simulink model "PLANTA_CODESYS"  (R2024b)
settings: Solver=FixedStepAuto  StartTime=0.0  StopTime=inf  FixedStep=0.001  MaxStep=0.0005  RelTol=1e-4
undefined symbols (not defined in the file): A_hm, A_tm, at_breakpoints, b_ha, B_hm, b_ta, B_tm, bcx, bcy, bhd, bhEb, bhm, bt, btd, btm, btw, bwu, C_hm, C_tm, D_hm, D_tm, DiscIntNeverNeededParam, dl_h_ini, dx_l_ini, dx_t_ini, dx_td_ini, dxt_max, dy_l_ini, g, Hc, ih, it, J_eqt, Jhd_hEb, Jhm_hb, Jtd, Jtm_tb, K_hsa, K_hsia, K_tsa, K_tsia, Kcy, Kd_table, ke_int, Ke_tita, ke_tita, ke_w, Ke_w, kp_pos, Kp_table, kp_w, kpos, Ktw, kwu, l_breakpoints, l_h_ini, Lh0, ml_breakpoints, Ms, Mt ... (+16)
libraries: simulink x11, spsEdgeDetectorLib x5, simulink_extras x2, opcualib x2, dspsigops x2, dspstat3 x1, vrlib x1, sldrtlib x1
(part 1 of 2)
settings Model: Creator=ribei  LastModifiedBy=ribei
settings SolverCC: AllowMultiTaskInputOutput=on  ZeroCrossAlgorithm=Adaptive  AutoInsertRateTranBlk=on
settings DebuggingCC: IgnoredZcDiagnostic=none  UnderSpecifiedDimensionMsg=warning

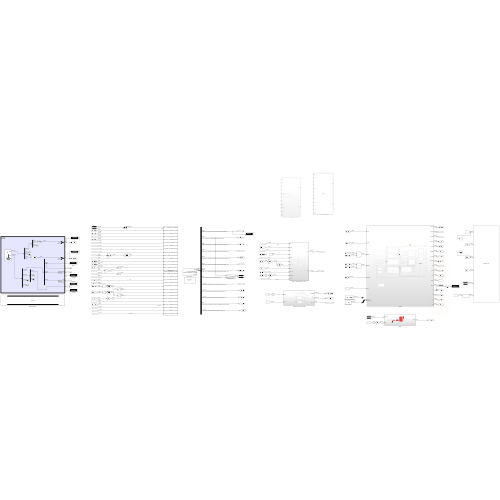
[thumbnail: Simulink's stored preview of the top-level diagram]
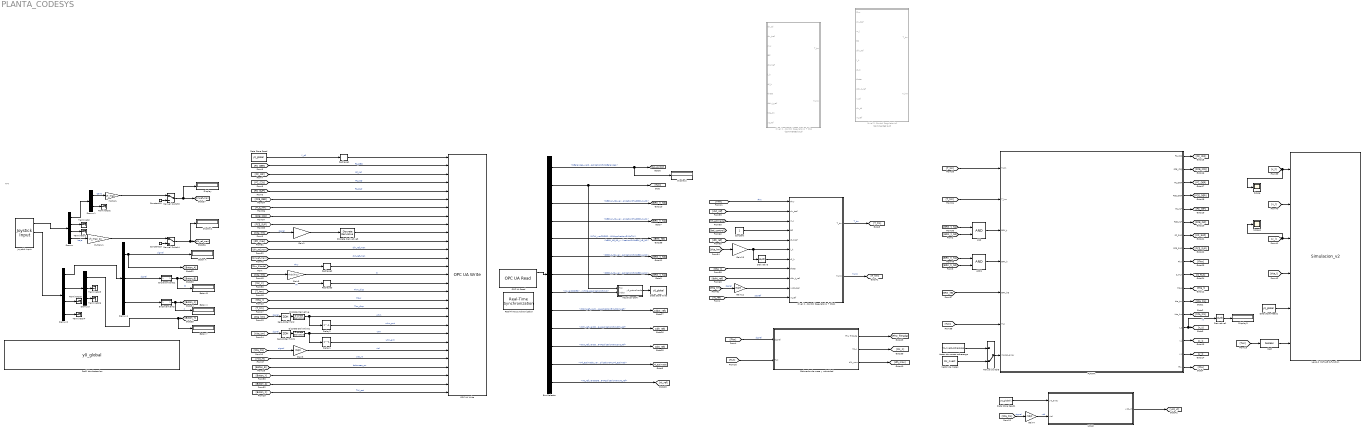
== system PLANTA_CODESYS ==
  note: HMI
  AND : Logic  IconShape=distinctive  AllPortsSameDT=off  OutDataTypeStr=boolean
  AND1 : Logic  IconShape=distinctive  AllPortsSameDT=off  OutDataTypeStr=boolean
  Actualizar perfil : Subsystem
  Boton A : Display
  Boton B : Display
  Boton X : Display
  Boton Y : Display
  Bus Selector : BusSelector  OutputSignals=bBalanceo_varCODESYSControlWinV3X64ApplicationGVLbBalanceo,bTLK_varCODESYSControlWinV3X64ApplicationGVLbTLK,bBRK_h_N0_varCODESYSControlWinV3X64ApplicationGVLbBRK_h_N0,bBRK_h_N1_varCODESYSControlWinV3X64ApplicationGVLbBRK_h_N1,bBRK_hE_N0_varCODESYSControlWinV3X64ApplicationGVLbBRK_hE_N0,bBRK_t_N0_varCODESYSControlWinV3X64ApplicationGVLbBRK_t_N0,bBRK_t_N1_varCODESYSControlWinV3X64ApplicationGVLbBRK_t_N1,iC_varCODESYSControlWinV3X64ApplicationGVLiC,rDdxt_ref_varCODESYSControlWinV3X64ApplicationGVLrDdxt_ref,rDlh_ref_varCODESYSControlWinV3X64ApplicationGVLrDlh_ref,rDxt_ref_varCODESYSControlWinV3X64ApplicationGVLrDxt_ref,rMl_estimada_varCODESYSControlWinV3X64ApplicationGVLrMl_estimad,rXt_ref_varCODESYSControlWinV3X64ApplicationGVLrXt_ref
  Cast : DataTypeConversion  OutDataTypeStr=boolean  SaturateOnIntegerOverflow=off  RndMeth=Floor
  Constant : Constant
  Constant18 : Constant  Value=0  SampleTime=T_s1
  Constant19 : Constant  Value=0  SampleTime=T_s1
  Data Store Read : DataStoreRead  DataStoreName=y0_global  IndexOptions=Index vector (dialog)  Indices=1  OutputSizes=1
  Data Store Read1 : DataStoreRead  DataStoreName=y0_global  DataStoreElements=y0_global(:)  IndexOptions=Index vector (dialog)  Indices=1  OutputSizes=1
  Data Store Read2 : DataStoreRead  DataStoreName=y0_global  IndexOptions=Index vector (dialog)  Indices=1  OutputSizes=1
  Data Store Write : DataStoreWrite  DataStoreName=y0_global  IndexOptions=Index vector (dialog)  Indices=1  OutputSizes=1
  Delay1 : Delay  DelayLength=1  InputProcessing=Columns as channels (frame based)  SampleTime=T_s1
  Delay2 : Delay  DelayLength=1  InputProcessing=Columns as channels (frame based)  SampleTime=T_s1
  Demux : Demux
  Demux1 : Demux  Outputs=2
  Demux2 : Demux
  Demux3 : Demux  Outputs=3
  Demux4 : Demux  Outputs=3
  Derivative : Derivative
  Derivative1 : Derivative
  Discrete Derivative : simulink/Discrete/Discrete Derivative  gainval=1.0  ICPrevScaledInput=0.0  OutMin=[]  OutMax=[]  OutDataType=fixdt(1, 16)  OutScaling=2^-10  DoSatur=off
  Discrete Derivative1 : simulink/Discrete/Discrete Derivative  gainval=1.0  ICPrevScaledInput=0.0  OutMin=[]  OutMax=[]  OutDataType=fixdt(1, 16)  OutScaling=2^-10  DoSatur=off
  Discrete Derivative3 : simulink/Discrete/Discrete Derivative  gainval=1.0  ICPrevScaledInput=0.0  OutMin=[]  OutMax=[]  OutDataType=fixdt(1, 16)  OutScaling=2^-10  DoSatur=off
  Display{,1..3} (4 alike) : Display
  Enclavamiento : Stateflow chart  TreatAsAtomicUnit=on
  Enclavamiento1 : Stateflow chart  TreatAsAtomicUnit=on
  Estimador de masa y velocidad : Subsystem
  Gain1 : Gain  Gain=-rhd/(ih*2)
  Gain12 : Gain  Gain=rtd/it
  Gain13 : Gain  Gain=-rhd/(ih*2)
  Gain3 : Gain  Gain=rtd/it
  Gain4 : Gain  Gain=rtd/it
  Gain5 : Gain  Gain=-rhd/(ih*2)
  Joystick Input : vrlib/Joystick Input  joyid=1  adjustports=on  forcefeed=off
  LIDAR : Subsystem
  Level-2 MATLAB S-Function : M-S-Function  FunctionName=Simulacion_v2  Parameters=2.438, 2.591, 1.500, 0.850, 0.750, 7.500, 2.100, 2.500, 'black', 'black', '#E99000', 5.000
  Manual Switch3 : ManualSwitch
  Manual Switch4 : ManualSwitch
  Manual Switch5 : ManualSwitch  CurrentSetting=0
  Multiply : Gain  Gain=vt_max
  Multiply1 : Gain  Gain=vh_max_sc
  Nivel 2 - Control Regulatorio + Obs : Subsystem  Commented=on
  Nivel 2 - Control Regulatorio + Obs1 : Subsystem
  Nivel 2: Control Regulatorio1 : MATLAB Function  Commented=on  TreatAsAtomicUnit=on  SystemSampleTime=T_s2
  OPC UA Read : opcualib/OPC UA Read  SelectedServer=OPCUAServer@DESKTOP-L47GKVF  ServerList=OPCUAServer@DESKTOP-L47GKVF  NodeList={ '1', 'bBalanceo', '4', '|var|CODESYS Control Win V3 x64.Application.GVL.bBalanceo', '0'; '2', 'bBRK_h_N0', '4', '|var|CODESYS Control Win V3 x64.Application.GVL.bBRK_h_N0', '0'; '3', 'bBRK_h_N1', '4', '|var|CODESYS Control Win V3 x64.Application.GVL.bBRK_h_N1', '0'; '4', 'bBRK_hE_N0', '4', '|var|CODESYS Control Win V3 x64.Application.GVL.bBRK_hE_N0', '0'; '5', 'bBRK_t_N0', '4', '|var|CODESYS Control Win V3 x64.Application.GVL.bBRK_t_N0', '0'; '6', 'bBRK_t_N1', '4', '|var|CODESYS Control Win V3 x64.Application.GVL.bBRK_t_N1', '0'; '7', 'bTLK', '4', '|var|CODESYS Control Win V3 x64.Application.GVL.bTLK', '0'; '8', 'iC', '4', '|var|CODESYS Control Win V3 x64.Application.GVL.iC', '0'; '9', 'rDdxt_ref', '4', '|var|CODESYS Control Win V3 x64.Application.GVL.rDdxt_ref', '0'; '10', 'rDlh_ref', '4', '|var|CODESYS Control Win V3 x64.Application.GVL.rDlh_ref', '0'; '11', 'rDxt_ref', '4', '|var|CODESYS Control Win V3 x64.Application.GVL.rDxt_ref', '0'; '12', 'rMl_estimada', '4', '|var|CODESYS Control Win V3 x64.Application.GVL.rMl_estimada', '0'; '13', 'rXt_ref', '4', '|var|CODESYS Control Win V3 x64.Application.GVL.rXt_ref', '0' }  ShowQualityPort=on  ShowTimestampPort=on  ShowTimestampPortAs=Seconds since start  SampleTime=T_s1
  OPC UA Write : opcualib/OPC UA Write  SelectedServer=OPCUAServer@DESKTOP-L47GKVF  ServerList=OPCUAServer@DESKTOP-L47GKVF  SampleTime=T_s1  NodeList={ '1', 'aY_c0', '4', '|var|CODESYS Control Win V3 x64.Application.GVL.aY_c0', '0'; '2', 'bFC_DER', '4', '|var|CODESYS Control Win V3 x64.Application.GVL.bFC_DER', '0'; '3', 'bFC_INF', '4', '|var|CODESYS Control Win V3 x64.Application.GVL.bFC_INF', '0'; '4', 'bFC_IZQ', '4', '|var|CODESYS Control Win V3 x64.Application.GVL.bFC_IZQ', '0'; '5', 'bFC_SUP', '4', '|var|CODESYS Control Win V3 x64.Application.GVL.bFC_SUP', '0'; '6', 'bFCE_DER', '4', '|var|CODESYS Control Win V3 x64.Application.GVL.bFCE_DER', '0'; '7', 'bFCE_INF', '4', '|var|CODESYS Control Win V3 x64.Application.GVL.bFCE_INF', '0'; '8', 'bFCE_IZQ', '4', '|var|CODESYS Control Win V3 x64.Application.GVL.bFCE_IZQ', '0'; '9', 'bFCE_SUP', '4', '|var|CODESYS Control Win V3 x64.Application.GVL.bFCE_SUP', '0'; '10', 'rDLh', '4', '|var|CODESYS Control Win V3 x64.Application.GVL.rDLh', '0'; '11', 'rDLh_max', '4', '|var|CODESYS Control Win V3 x64.Application.GVL.rDLh_max', '0'; '12', 'rDLh_ref_man', '4', '|var|CODESYS Control Win V3 x64.Application.GVL.rDLh_ref_man', '0'; '13', 'rDXt_ref_man', '4', '|var|CODESYS Control Win V3 x64.Application.GVL.rDXt_ref_man', '0'; '14', 'rFhw', '4', '|var|CODESYS Control Win V3 x64.Application.GVL.rFhw', '0'; '15', 'rLh', '4', '|var|CODESYS Control Win V3 x64.Application.GVL.rLh', '0'; '16', 'rMl', '4', '|var|CODESYS Control Win V3 x64.Application.GVL.rMl', '0'; '17', 'rThm_disp', '4', '|var|CODESYS Control Win V3 x64.Application.GVL.rThm_disp', '0'; '18', 'rTita_l', '4', '|var|CODESYS Control Win V3 x64.Application.GVL.rTita_l', '0'; '19', 'rTtm_disp', '4', '|var|CODESYS Control Win V3 x64.Application.GVL.rTtm_disp', '0'; '20', 'rWhm', '4', '|var|CODESYS Control Win V3 x64.Application.GVL.rWhm', '0'; '21', 'rWhm_ant', '4', '|var|CODESYS Control Win V3 x64.Application.GVL.rWhm_ant', '0'; '22', 'rWtm', '4', '|var|CODESYS Control Win V3 x64.Application.GVL.rWtm', '0'; '23', 'rWtm_ant', '4', '|var|CODESYS Control Win V3 x64.Application.GVL.rWtm_ant', '0'; '24', 'rXtd', '4', '|var|CODESYS Control Win V3 x64.Application.GVL.rXtd', '0'; '25', 'rYc0_xt', '4', '|var|CODESYS Control Win V3 x64.Application.GVL.rYc0_xt', '0'; '26', 'pBAL_ON', '4', '|var|CODESYS Control Win V3 x64.Application.GVL.pBAL_ON', '0'; '27', 'pP_EM', '4', '|var|CODESYS Control Win V3 x64.Application.GVL.pP_EM', '0'; '28', 'pP_OK', '4', '|var|CODESYS Control Win V3 x64.Application.GVL.pP_OK', '0'; '29', 'pTLK_ACT', '4', '|var|CODESYS Control Win V3 x64.Application.GVL.pTLK_ACT', '0' }
  PLANTA : Subsystem
  Perfil de obstaculos : DataStoreMemory  DataStoreName=y0_global  WriteAfterWriteMsg=warning  InitialValue=y0  ShowAdditionalParam=off  OutDataTypeStr=double
  Real-Time Synchronization : sldrtlib/Real-Time Synchronization  SampleTime=0.02  MaxMissedTicks=10  ShowMissedTicks=off  YieldWhenWaiting=on
  Reshape1 : Reshape  OutputDimensionality=Row vector (2-D)
  Reshape2 : Reshape
  Reshape3 : Reshape
  Scope : Scope
  Scope1 : Scope
  Terminator{,1..6} (7 alike) : Terminator
  Vector de masas : FromWorkspace  VariableName=Mc_Xvect
  Vector de masas sobrecarga : FromWorkspace  VariableName=Mc_Xvect_sobrecarga
  Zero-Order Hold : ZeroOrderHold  SampleTime=T_s1
  Zero-Order Hold1 : ZeroOrderHold  SampleTime=T_s1
  wires:
  PLANTA/12(tita_tm) -> [tita_tm]
  PLANTA/13(tita_hm) -> [tita_hm]
  PLANTA/14(x_t) -> Derivative1/1, [x_t]  "xt"
  PLANTA/15(x_l) -> [x_l]
  PLANTA/16(y_l) -> [y_l]
  Data Store Read2/1 -> Level-2 MATLAB S-Function/5
  [tita_l] -> Level-2 MATLAB S-Function/4
  Gain3/1 -> OPC UA Write/24  "xtd"
  [tita_hm] -> Zero-Order Hold/1  "signal"
  [tita_tm] -> Zero-Order Hold1/1  "signal"
  Gain5/1 -> OPC UA Write/15  "lh"
  Demux4/1 -> Boton A/1, [Boton_A]  "signal"
  Demux4/2 -> Enclavamiento1/1(input)  "signal"
  [T_tm] -> PLANTA/1(T_tm)
  [T_hm] -> PLANTA/2(T_hm)
  [BRK_hE] -> PLANTA/5(BRK_hE)
  [TLK] -> PLANTA/6(TLK)
  PLANTA/11(tita_l) -> [tita_l]
  [x_t] -> Scope/1, Level-2 MATLAB S-Function/1
  [x_l] -> Level-2 MATLAB S-Function/2
  [y_l] -> Scope1/1, Level-2 MATLAB S-Function/3
  PLANTA/1(FC_IZQ) -> [FC_IZQ]
  PLANTA/2(FCE_IZQ) -> [FCE_IZQ]
  PLANTA/3(FC_DER) -> [FC_DER]
  PLANTA/4(FCE_DER) -> [FCE_DER]
  PLANTA/5(FC_INF) -> [FC_INF]
  PLANTA/6(FCE_INF) -> [FCE_INF]
  PLANTA/7(FC_SUP) -> [FC_SUP]
  PLANTA/8(FCE_SUP) -> [FCE_SUP]
  PLANTA/9(Fhw) -> [Fhw]
  PLANTA/10(S_TLK) -> [S_TLK]
  [tita_tm] -> Gain3/1  "signal"
  Discrete Derivative1/1 -> OPC UA Write/22, Delay1/1  "wtm"
  [tita_hm] -> Gain5/1
  Actualizar perfil/1(y0_actualizado) -> Data Store Write/1
  PLANTA/17(Ftw) -> [Ftw]
  Demux/1 -> Demux1/1
  Demux/3 -> Terminator1/1
  Demux1/2 -> Terminator2/1
  Demux/2 -> Terminator/1
  Joystick Input/1 -> Demux/1
  Constant18/1 -> Manual Switch3/2
  Demux1/1 -> Multiply/1  "Carro"
  Constant19/1 -> Manual Switch4/2
  Demux/4 -> Multiply1/1  "Izaje"
  Demux3/1 -> Boton Y/1, [Boton_Y]
  Demux3/2 -> Terminator5/1
  Demux4/3 -> Enclavamiento/1(input)
  Demux2/2 -> Demux3/1
  Demux2/4 -> Terminator4/1
  Demux3/3 -> Terminator6/1
  Joystick Input/2 -> Demux2/1
  Demux2/3 -> Terminator3/1
  Demux2/1 -> Demux4/1
  Multiply1/1 -> Manual Switch4/1
  Discrete Derivative/1 -> OPC UA Write/20, Delay2/1  "whm"
  Delay1/1 -> OPC UA Write/23  "wtm_ant"
  Zero-Order Hold/1 -> Discrete Derivative/1
  Zero-Order Hold1/1 -> Discrete Derivative1/1
  [T_tm] -> OPC UA Write/19  "Ttm_disp"
  [T_hm] -> OPC UA Write/17  "Thm_disp"
  [TLK] -> Cast/1
  Delay2/1 -> OPC UA Write/21  "whm_ant"
  Multiply/1 -> Manual Switch3/1
  [tita_l] -> OPC UA Write/18  "tita_l"
  Manual Switch5/1 -> PLANTA/7(masas_array)
  Vector de masas/1 -> Manual Switch5/2
  Vector de masas sobrecarga/1 -> Manual Switch5/1
  [Boton_B] -> OPC UA Write/26  "balanceo_on"
  [Boton_X] -> OPC UA Write/29  "TLK_act"
  Enclavamiento1/1(output) -> Boton B/1, [Boton_B]  "B"
  Enclavamiento/1(output) -> Boton X/1, [Boton_X]  "X"
  Manual Switch4/1 -> Display1/1, [dlh_ref_man]
  Manual Switch3/1 -> Display/1, [dxt_ref_man]
  [dlh_ref_man] -> OPC UA Write/12  "dlh_ref_man"
  [dxt_ref_man] -> OPC UA Write/13  "dxt_ref_man"
  [Fhw] -> Estimador de masa y velocidad/1(signal)  "signal"
  [TLK] -> Estimador de masa y velocidad/2(TLK)
  Estimador de masa y velocidad/1(Fhw filtrada) -> [Fhw_filtrada]
  Estimador de masa y velocidad/2(Mc_x) -> [Mc_X]
  Estimador de masa y velocidad/3(dlh_max) -> [dlh_max]
  Data Store Read1/1 -> LIDAR/1(y0_array)
  [tita_tm] -> Gain4/1  "signal"
  Gain4/1 -> LIDAR/2(xtd)  "xtd"
  LIDAR/1(yc0_xt) -> [yc0_xt]
  [Mc_X] -> Reshape3/1  "Ml"
  [Fhw_filtrada] -> Reshape2/1  "Fhw"
  [FC_SUP] -> OPC UA Write/5  "FC_SUP"
  [FC_INF] -> OPC UA Write/3  "FC_INF"
  [FC_IZQ] -> OPC UA Write/4  "FC_IZQ"
  [FC_DER] -> OPC UA Write/2  "FC_DER"
  [yc0_xt] -> OPC UA Write/25  "yc0_xt"
  Data Store Read/1 -> Reshape1/1  "Y_c0"
  Reshape1/1 -> OPC UA Write/1
  Reshape2/1 -> OPC UA Write/14
  Reshape3/1 -> OPC UA Write/16
  [tita_hm] -> Gain1/1  "signal"
  [Boton_A] -> OPC UA Write/28
  [Boton_Y] -> OPC UA Write/27
  [FCE_DER] -> OPC UA Write/6
  [FCE_INF] -> OPC UA Write/7
  [FCE_IZQ] -> OPC UA Write/8
  [FCE_SUP] -> OPC UA Write/9
  Cast/1 -> Level-2 MATLAB S-Function/6
  OPC UA Read/1 -> Bus Selector/1
  Bus Selector/1 -> [bal_control], Display2/1  "<bBalanceo_varCODESYSControlWinV3X64ApplicationGVLbBalanceo>"
  Bus Selector/2 -> [TLK], Actualizar perfil/1(TLK)  "<bTLK_varCODESYSControlWinV3X64ApplicationGVLbTLK>"
  Bus Selector/8 -> Actualizar perfil/2(index)  "<iC_varCODESYSControlWinV3X64ApplicationGVLiC>"
  Bus Selector/9 -> [ddxt_ref]  "<rDdxt_ref_varCODESYSControlWinV3X64ApplicationGVLrDdxt_ref>"
  Bus Selector/10 -> [dlh_ref]  "<rDlh_ref_varCODESYSControlWinV3X64ApplicationGVLrDlh_ref>"
  Bus Selector/11 -> [dxt_ref]  "<rDxt_ref_varCODESYSControlWinV3X64ApplicationGVLrDxt_ref>"
  Bus Selector/12 -> [Ml_estimada]  "<rMl_estimada_varCODESYSControlWinV3X64ApplicationGVLrMl_estimad>"
  Nivel 2 - Control Regulatorio + Obs1/1(T_tm) -> [T_tm]  "T_tm"
  [tita_hm] -> Gain13/1
  Nivel 2 - Control Regulatorio + Obs1/2(T_hm) -> [T_hm]  "T_hm"
  [tita_tm] -> Gain12/1  "signal"
  [BRK_t_N0] -> AND/2
  [BRK_t_N1] -> AND/1
  AND/1 -> PLANTA/3(BRK_t)
  [BRK_h_N0] -> AND1/2
  [BRK_h_N1] -> AND1/1
  AND1/1 -> PLANTA/4(BRK_h)
  Bus Selector/3 -> [BRK_h_N0]  "<bBRK_h_N0_varCODESYSControlWinV3X64ApplicationGVLbBRK_h_N0>"
  Bus Selector/4 -> [BRK_h_N1]  "<bBRK_h_N1_varCODESYSControlWinV3X64ApplicationGVLbBRK_h_N1>"
  Bus Selector/5 -> [BRK_hE]  "<bBRK_hE_N0_varCODESYSControlWinV3X64ApplicationGVLbBRK_hE_N0>"
  Bus Selector/6 -> [BRK_t_N0]  "<bBRK_t_N0_varCODESYSControlWinV3X64ApplicationGVLbBRK_t_N0>"
  Bus Selector/7 -> [BRK_t_N1]  "<bBRK_t_N1_varCODESYSControlWinV3X64ApplicationGVLbBRK_t_N1>"
  Bus Selector/13 -> [xt_ref]  "<rXt_ref_varCODESYSControlWinV3X64ApplicationGVLrXt_ref>"
  [dlh_max] -> OPC UA Write/11
  [Ml_estimada] -> Nivel 2 - Control Regulatorio + Obs1/3(m_l)
  Gain13/1 -> Nivel 2 - Control Regulatorio + Obs1/6(l_h), Derivative/1
  [tita_l] -> Nivel 2 - Control Regulatorio + Obs1/8(theta)
  Gain12/1 -> Nivel 2 - Control Regulatorio + Obs1/10(x_td_real)
  [Fhw] -> Nivel 2 - Control Regulatorio + Obs1/1(Fhw)  "Fhw"
  Gain1/1 -> Discrete Derivative3/1
  Discrete Derivative3/1 -> OPC UA Write/10
  Derivative/1 -> Nivel 2 - Control Regulatorio + Obs1/7(dl_h)
  Constant/1 -> Nivel 2 - Control Regulatorio + Obs1/4(BC)
  [xt_ref] -> Nivel 2 - Control Regulatorio + Obs1/11(xt_ref)  "posref"
  [ddxt_ref] -> Nivel 2 - Control Regulatorio + Obs1/9(ddx_t_ref)
  [dxt_ref] -> Nivel 2 - Control Regulatorio + Obs1/2(dx_tref)
  [dlh_ref] -> Nivel 2 - Control Regulatorio + Obs1/5(dl_href)
  Derivative1/1 -> Display3/1

== system PLANTA_CODESYS/Actualizar perfil ==
  TLK : Inport
  index : Inport  Port=2
  Data Store Read3 : DataStoreRead  DataStoreName=y0_global  IndexOptions=Index vector (dialog)  Indices=1  OutputSizes=1
  Edge Detector1 : spsEdgeDetectorLib/Edge Detector  model=Either  ic=0  Ts=-1
      settings: LibrarySourceBlock=sps_lib/Control/Edge Detector
  Enabled Subsystem : Subsystem  TreatAsAtomicUnit=on
  Switch : Switch  Criteria=u2 > Threshold  SaturateOnIntegerOverflow=off  InputSameDT=off
  Unit Delay : UnitDelay  SampleTime=-1  HasFrameUpgradeWarning=on
  y0_actualizado : Outport
  wires:
  Unit Delay/1 -> Edge Detector1/1
  TLK/1 -> Unit Delay/1
  Edge Detector1/1 -> Switch/2, Enabled Subsystem/Enable
  Enabled Subsystem/1(y0_actualizado) -> Switch/1
  index/1 -> Enabled Subsystem/1(index)
  Switch/1 -> y0_actualizado/1
  Data Store Read3/1 -> Switch/3

== system PLANTA_CODESYS/Estimador de masa y velocidad ==
  signal : Inport
  TLK : Inport  Port=2
  Constant9 : Constant  Value=Ms
  Masa contenedor : Subsystem
  Moving Average : dspstat3/Moving Average  Method=Sliding window  ForgettingFactorPort=off  SpecifyWindowLength=on  WindowLength=40  OverlapLength=0  AllowArbitraryInputLength=off  ForgettingFactor=0.9  SimulateUsing=Interpreted execution
  Sum1 : Sum  Inputs=|++
  Tapped Delay : simulink/Discrete/Tapped Delay  vinit=0.0  samptime=T_s1  NumDelays=40  DelayOrder=Oldest  includeCurrent=off
  Velocidad max izaje : MATLAB Function  TreatAsAtomicUnit=on
  Zero-Order Hold2 : ZeroOrderHold  SampleTime=T_s1
  Fhw filtrada : Outport
  Mc_x : Outport  Port=2
  dlh_max : Outport  Port=3
  wires:
  Tapped Delay/1 -> Moving Average/1
  Sum1/1 -> Velocidad max izaje/1(M_l)
  Masa contenedor/1(Mc_X) -> Mc_x/1, Sum1/1  "Mc_x"
  Constant9/1 -> Sum1/2
  Moving Average/1 -> Fhw filtrada/1, Masa contenedor/1(Fwh)  "Fhw filtrada"
  Zero-Order Hold2/1 -> Tapped Delay/1  "señal cruda"
  Velocidad max izaje/1(dxt_max) -> dlh_max/1  "dlh_max"
  signal/1 -> Zero-Order Hold2/1
  TLK/1 -> Masa contenedor/2(TLK)

== system PLANTA_CODESYS/LIDAR ==
  y0_array : Inport
  xtd : Inport  Port=2
  Ajuste referencia : Constant  Value=30
  Constant15 : Constant  Value=Yt0
  Data Type Conversion : DataTypeConversion  OutDataTypeStr=int32  RndMeth=Ceiling  SaturateOnIntegerOverflow=off
  Gain : Gain  Gain=1/Wc
  Sum : Sum  Inputs=|++
  Sum2 : Sum  Inputs=+-|
  sensor : MATLAB Function  TreatAsAtomicUnit=on
  yc0_xt : Outport
  wires:
  Sum/1 -> Gain/1
  xtd/1 -> Sum/1
  Gain/1 -> Data Type Conversion/1
  Ajuste referencia/1 -> Sum/2
  Constant15/1 -> Sum2/1
  Data Type Conversion/1 -> sensor/2(index)
  y0_array/1 -> sensor/1(y0_array)
  sensor/1(distancia) -> Sum2/2
  Sum2/1 -> yc0_xt/1

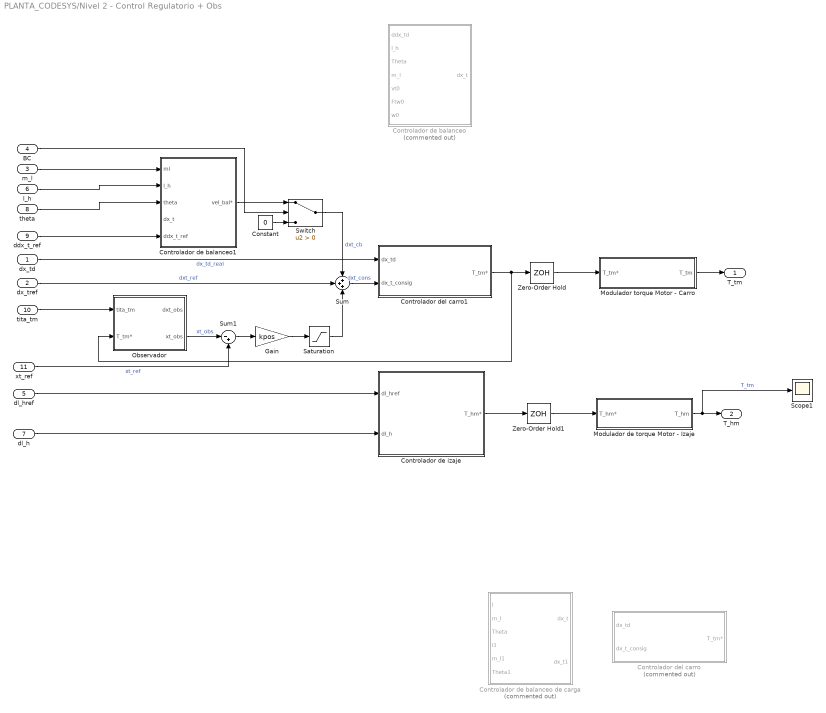
== system PLANTA_CODESYS/Nivel 2 - Control Regulatorio + Obs ==
  dx_td : Inport
  dx_tref : Inport  Port=2
  m_l : Inport  Port=3
  BC : Inport  Port=4
  dl_href : Inport  Port=5
  l_h : Inport  Port=6
  dl_h : Inport  Port=7
  theta : Inport  Port=8
  ddx_t_ref : Inport  Port=9
  tita_tm : Inport  Port=10
  xt_ref : Inport  Port=11
  Constant : Constant  Value=0
  Controlador de balanceo : Subsystem  Commented=on
  Controlador de balanceo de carga : Subsystem  Commented=on
  Controlador de balanceo1 : Subsystem
  Controlador de izaje : Subsystem
  Controlador del carro : Subsystem  Commented=on
  Controlador del carro1 : Subsystem
  Gain : Gain  Gain=kpos
  Modulador de torque Motor - Izaje : Subsystem
  Modulador torque Motor - Carro : Subsystem
  Observador : Subsystem
  Saturation : Saturate  UpperLimit=dxt_max  LowerLimit=-dxt_max
  Scope1 : Scope
  Sum : Sum  Inputs=+++
  Sum1 : Sum  Inputs=|-+
  Switch : Switch  Criteria=u2 > Threshold  SaturateOnIntegerOverflow=off  InputSameDT=off
  Zero-Order Hold : ZeroOrderHold  SampleTime=T_s2
  Zero-Order Hold1 : ZeroOrderHold  SampleTime=T_s2
  T_tm : Outport
  T_hm : Outport  Port=2
  wires:
  dl_href/1 -> Controlador de izaje/1(dl_href)
  Zero-Order Hold1/1 -> Modulador de torque Motor - Izaje/1(T_hm*)
  dl_h/1 -> Controlador de izaje/2(dl_h)
  Controlador de izaje/1(T_hm*) -> Zero-Order Hold1/1
  Modulador de torque Motor - Izaje/1(T_hm) -> Scope1/1, T_hm/1  "T_tm"
  Zero-Order Hold/1 -> Modulador torque Motor - Carro/1(T_tm*)
  Modulador torque Motor - Carro/1(T_tm) -> T_tm/1
  l_h/1 -> Controlador de balanceo1/2(l_h)
  Constant/1 -> Switch/3
  m_l/1 -> Controlador de balanceo1/1(ml)
  BC/1 -> Switch/2
  Controlador del carro1/1(T_tm*) -> Observador/2(T_tm*), Zero-Order Hold/1
  Controlador de balanceo1/1(vel_bal*) -> Switch/1
  theta/1 -> Controlador de balanceo1/3(theta)
  dx_tref/1 -> Sum/2  "dxt_ref"
  Sum/1 -> Controlador del carro1/2(dx_t_consig)  "dxt_cons"
  Switch/1 -> Sum/1  "dxt_cb"
  ddx_t_ref/1 -> Controlador de balanceo1/5(ddx_t_ref)
  tita_tm/1 -> Observador/1(tita_tm)
  Observador/2(xt_obs) -> Sum1/1  "xt_obs"
  xt_ref/1 -> Sum1/2  "xt_ref"
  Sum1/1 -> Gain/1
  dx_td/1 -> Controlador del carro1/1(dx_td)  "dx_td_real"
  Gain/1 -> Saturation/1
  Saturation/1 -> Sum/3

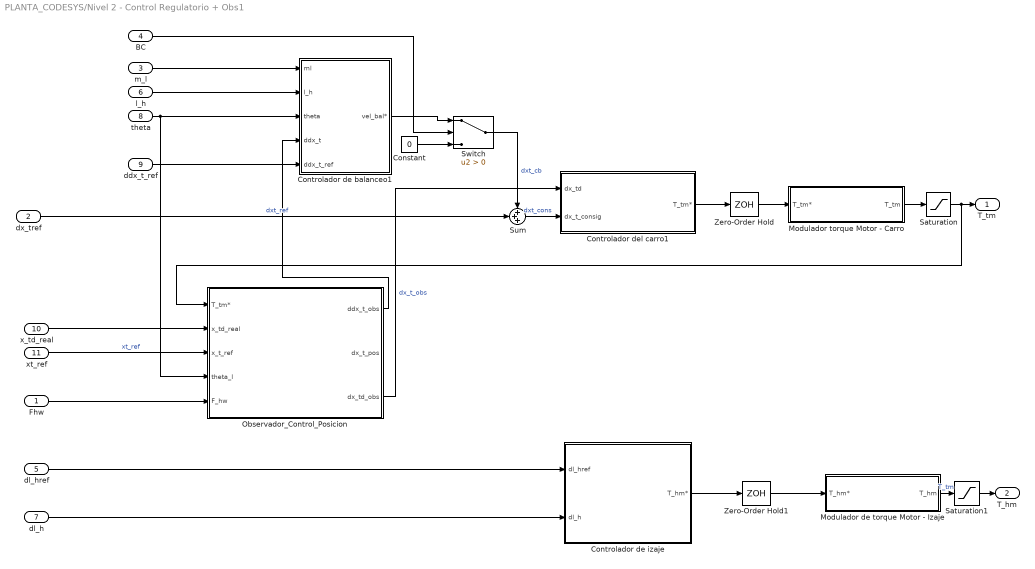
== system PLANTA_CODESYS/Nivel 2 - Control Regulatorio + Obs1 ==
  Fhw : Inport
  dx_tref : Inport  Port=2
  m_l : Inport  Port=3
  BC : Inport  Port=4
  dl_href : Inport  Port=5
  l_h : Inport  Port=6
  dl_h : Inport  Port=7
  theta : Inport  Port=8
  ddx_t_ref : Inport  Port=9
  x_td_real : Inport  Port=10
  xt_ref : Inport  Port=11
  Constant : Constant  Value=0
  Controlador de balanceo1 : Subsystem
  Controlador de izaje : Subsystem
  Controlador del carro1 : Subsystem
  Modulador de torque Motor - Izaje : Subsystem
  Modulador torque Motor - Carro : Subsystem
  Observador_Control_Posicion : Subsystem
  Saturation : Saturate  UpperLimit=3000  LowerLimit=3000
  Saturation1 : Saturate  UpperLimit=3000  LowerLimit=3000
  Sum : Sum  Inputs=+++
  Switch : Switch  Criteria=u2 > Threshold  SaturateOnIntegerOverflow=off  InputSameDT=off
  Zero-Order Hold : ZeroOrderHold  SampleTime=T_s2
  Zero-Order Hold1 : ZeroOrderHold  SampleTime=T_s2
  T_tm : Outport
  T_hm : Outport  Port=2
  wires:
  Zero-Order Hold1/1 -> Modulador de torque Motor - Izaje/1(T_hm*)
  Controlador de izaje/1(T_hm*) -> Zero-Order Hold1/1
  Modulador de torque Motor - Izaje/1(T_hm) -> Saturation1/1  "T_tm"
  Zero-Order Hold/1 -> Modulador torque Motor - Carro/1(T_tm*)
  l_h/1 -> Controlador de balanceo1/2(l_h)
  Constant/1 -> Switch/3
  m_l/1 -> Controlador de balanceo1/1(ml)
  BC/1 -> Switch/2
  Controlador del carro1/1(T_tm*) -> Zero-Order Hold/1
  Controlador de balanceo1/1(vel_bal*) -> Switch/1
  theta/1 -> Controlador de balanceo1/3(theta), Observador_Control_Posicion/4(theta_l)
  dx_tref/1 -> Sum/2  "dxt_ref"
  Sum/1 -> Controlador del carro1/2(dx_t_consig)  "dxt_cons"
  Observador_Control_Posicion/3(dx_td_obs) -> Controlador del carro1/1(dx_td)  "dx_t_obs"
  Observador_Control_Posicion/1(ddx_t_obs) -> Controlador de balanceo1/4(ddx_t)
  xt_ref/1 -> Observador_Control_Posicion/3(x_t_ref)  "xt_ref"
  x_td_real/1 -> Observador_Control_Posicion/2(x_td_real)
  Fhw/1 -> Observador_Control_Posicion/5(F_hw)
  dl_h/1 -> Controlador de izaje/2(dl_h)
  ddx_t_ref/1 -> Controlador de balanceo1/5(ddx_t_ref)
  dl_href/1 -> Controlador de izaje/1(dl_href)
  Modulador torque Motor - Carro/1(T_tm) -> Saturation/1
  Switch/1 -> Sum/1  "dxt_cb"
  Saturation/1 -> Observador_Control_Posicion/1(T_tm*), T_tm/1
  Saturation1/1 -> T_hm/1

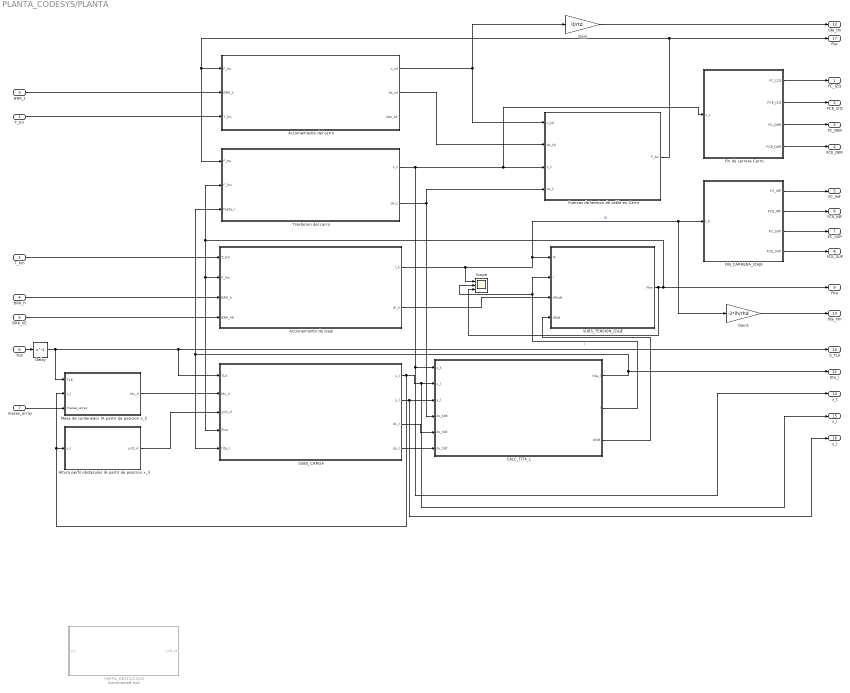
== system PLANTA_CODESYS/PLANTA ==
  T_tm : Inport
  T_hm : Inport  Port=2
  BRK_t : Inport  Port=3
  BRK_h : Inport  Port=4
  BRK_hE : Inport  Port=5
  TLK : Inport  Port=6
  masas_array : Inport  Port=7
  Accionamiento de Izaje : Subsystem
  Accionamiento del carro : Subsystem
  Altura perfil obstaculos (A partir de posicion x_l) : Subsystem
  CALC_TITA_L : Subsystem
  Delay : Delay  DelayLength=1  InputProcessing=Columns as channels (frame based)  SampleTime=T_s1
  FIN_CARRERA_IZAJE : Subsystem
  Fin de carrera Carro : Subsystem
  Fuerzas de tension de cable en Carro : Subsystem
  Gain : Gain  Gain=it/rtd
  Gain1 : Gain  Gain=-2*ih/rhd
  Masa de contenedor (A partir de posicion x_l) : Subsystem
  PERFIL_OBSTACULOS : Subsystem  Commented=on
  SUBS_CARGA : Subsystem
  SUBS_TENSION_IZAJE : Subsystem
  Scope : Scope  NumInputPorts=3
  Traslacion del carro : Subsystem
  FC_IZQ : Outport
  FCE_IZQ : Outport  Port=2
  FC_DER : Outport  Port=3
  FCE_DER : Outport  Port=4
  FC_INF : Outport  Port=5
  FCE_INF : Outport  Port=6
  FC_SUP : Outport  Port=7
  FCE_SUP : Outport  Port=8
  Fhw : Outport  Port=9
  S_TLK : Outport  Port=10
  tita_l : Outport  Port=11
  tita_tm : Outport  Port=12
  tita_hm : Outport  Port=13
  x_t : Outport  Port=14
  x_l : Outport  Port=15
  y_l : Outport  Port=16
  Ftw : Outport  Port=17
  wires:
  Gain/1 -> tita_tm/1
  Traslacion del carro/2(dx_t) -> CALC_TITA_L/4(dx_t/dt), Fuerzas de tension de cable en Carro/4(dx_t)
  SUBS_TENSION_IZAJE/1(Fhw) -> Scope/3, Fhw/1, Traslacion del carro/2(F_hw), Accionamiento de Izaje/2(F_hw), SUBS_CARGA/4(Fhw)
  CALC_TITA_L/3(dl/dt) -> SUBS_TENSION_IZAJE/4(dl/dt)
  BRK_h/1 -> Accionamiento de Izaje/3(BRK_h)
  TLK/1 -> Delay/1
  BRK_t/1 -> Accionamiento del carro/2(BRK_t)
  Accionamiento del carro/1(x_td) -> Fuerzas de tension de cable en Carro/1(x_td), Gain/1
  BRK_hE/1 -> Accionamiento de Izaje/4(BRK_hE)
  Accionamiento del carro/2(dx_td) -> Fuerzas de tension de cable en Carro/2(dx_td)
  FIN_CARRERA_IZAJE/3(FC_SUP) -> FC_SUP/1
  Fin de carrera Carro/4(FCE_DER) -> FCE_DER/1
  SUBS_CARGA/4(dy_l) -> CALC_TITA_L/6(dy_l/dt)
  CALC_TITA_L/2(l) -> SUBS_TENSION_IZAJE/2(l), Scope/2  "l"
  Fuerzas de tension de cable en Carro/1(F_tw) -> Ftw/1, Accionamiento del carro/1(F_tw), Traslacion del carro/1(F_tw)
  SUBS_CARGA/3(dx_l) -> CALC_TITA_L/5(dx_l/dt)
  Altura perfil obstaculos (A partir de posicion x_l)/1(yc0_xl) -> SUBS_CARGA/3(yc0_xl)
  Accionamiento de Izaje/1(l_h) -> SUBS_TENSION_IZAJE/1(Ih), FIN_CARRERA_IZAJE/1(l_h), Gain1/1, Scope/1  "lh"
  Accionamiento de Izaje/2(dl_h) -> SUBS_TENSION_IZAJE/3(dlh/dt)
  T_tm/1 -> Accionamiento del carro/3(T_tm)
  Fin de carrera Carro/2(FCE_IZQ) -> FCE_IZQ/1
  T_hm/1 -> Accionamiento de Izaje/1(T_hm)
  FIN_CARRERA_IZAJE/1(FC_INF) -> FC_INF/1
  Gain1/1 -> tita_hm/1
  FIN_CARRERA_IZAJE/2(FCE_INF) -> FCE_INF/1
  Fin de carrera Carro/1(FC_IZQ) -> FC_IZQ/1
  FIN_CARRERA_IZAJE/4(FCE_SUP) -> FCE_SUP/1
  Fin de carrera Carro/3(FC_DER) -> FC_DER/1
  SUBS_CARGA/1(x_l) -> Masa de contenedor (A partir de posicion x_l)/2(x_l), Altura perfil obstaculos (A partir de posicion x_l)/1(x_l), x_l/1, CALC_TITA_L/2(x_l)
  CALC_TITA_L/1(tita_l) -> tita_l/1, Traslacion del carro/3(theta_l), SUBS_CARGA/5(tita_l)
  Traslacion del carro/1(x_t) -> CALC_TITA_L/1(x_t), x_t/1, Fin de carrera Carro/1(x_t), Fuerzas de tension de cable en Carro/3(x_t)
  SUBS_CARGA/2(y_l) -> y_l/1, CALC_TITA_L/3(y_l)
  Masa de contenedor (A partir de posicion x_l)/1(Mc_X) -> SUBS_CARGA/2(Mc_X)
  Delay/1 -> Masa de contenedor (A partir de posicion x_l)/1(TLK), S_TLK/1, SUBS_CARGA/1(TLK)
  masas_array/1 -> Masa de contenedor (A partir de posicion x_l)/3(masas_array)

== system PLANTA_CODESYS/Actualizar perfil/Enabled Subsystem ==
  index : Inport
  Enable : EnablePort
  Actualiza perfil : MATLAB Function  TreatAsAtomicUnit=on
  Constant16 : Constant  Value=Hc
  Data Store Read3 : DataStoreRead  DataStoreName=y0_global  IndexOptions=Index vector (dialog)  Indices=1  OutputSizes=1
  y0_actualizado : Outport
  wires:
  Data Store Read3/1 -> Actualiza perfil/2(y0)
  Constant16/1 -> Actualiza perfil/3(Hc)
  index/1 -> Actualiza perfil/1(index)
  Actualiza perfil/1(y0_actualizado) -> y0_actualizado/1

== system PLANTA_CODESYS/Estimador de masa y velocidad/Masa contenedor ==
  Fwh : Inport
  TLK : Inport  Port=2
  Edge Detector : spsEdgeDetectorLib/Edge Detector  model=Falling  ic=0  Ts=-1
      settings: LibrarySourceBlock=sps_lib/Control/Edge Detector
  Edge Detector1 : spsEdgeDetectorLib/Edge Detector  model=Rising  ic=0  Ts=-1
      settings: LibrarySourceBlock=sps_lib/Control/Edge Detector
  Gain8 : Gain  Gain=2/g
  Product : Product
  S-R Flip-Flop : simulink_extras/Flip Flops/S-R Flip-Flop  initial_condition=0
  Unit Delay : UnitDelay  SampleTime=-1  HasFrameUpgradeWarning=on
  Mc_X : Outport
  wires:
  TLK/1 -> Unit Delay/1
  Edge Detector/1 -> S-R Flip-Flop/2
  Edge Detector1/1 -> S-R Flip-Flop/1
  S-R Flip-Flop/1 -> Product/2
  Product/1 -> Mc_X/1
  Unit Delay/1 -> Edge Detector1/1, Edge Detector/1
  Fwh/1 -> Gain8/1  "m estimada"
  Gain8/1 -> Product/1  "m estimada"

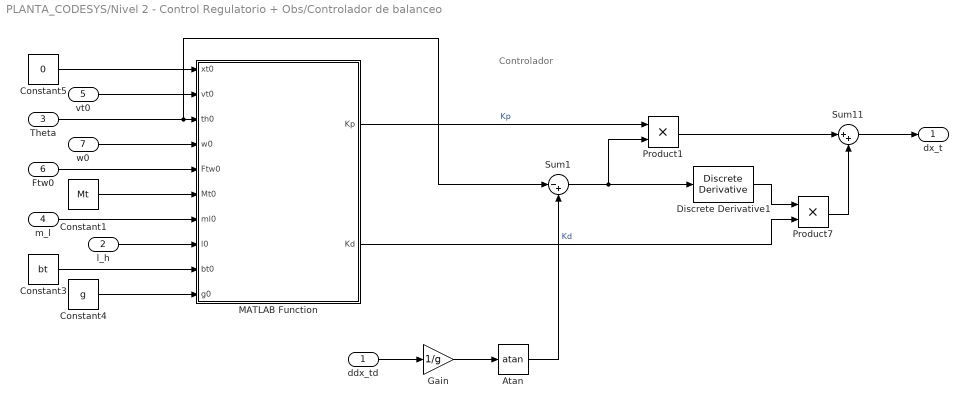
== system PLANTA_CODESYS/Nivel 2 - Control Regulatorio + Obs/Controlador de balanceo ==
  note: Controlador
  ddx_td : Inport
  l_h : Inport  Port=2
  Theta : Inport  Port=3
  m_l : Inport  Port=4
  vt0 : Inport  Port=5
  Ftw0 : Inport  Port=6
  w0 : Inport  Port=7
  Atan : Trigonometry  Operator=atan
  Constant1 : Constant  Value=Mt
  Constant3 : Constant  Value=bt
  Constant4 : Constant  Value=g
  Constant5 : Constant  Value=0
  Discrete Derivative1 : simulink/Discrete/Discrete Derivative  gainval=1.0  ICPrevScaledInput=0.0  OutMin=[]  OutMax=[]  OutDataType=fixdt(1, 16)  OutScaling=2^-10  DoSatur=off
  Gain : Gain  Gain=1/g
  MATLAB Function : MATLAB Function  TreatAsAtomicUnit=on
  Product1 : Product
  Product7 : Product
  Sum1 : Sum  Inputs=|-+
  Sum11 : Sum  Inputs=|++
  dx_t : Outport
  wires:
  Discrete Derivative1/1 -> Product7/1
  Sum11/1 -> dx_t/1
  MATLAB Function/2(Kd) -> Product7/2  "Kd"
  Product7/1 -> Sum11/2
  Constant1/1 -> MATLAB Function/6(Mt0)
  m_l/1 -> MATLAB Function/7(ml0)
  Constant3/1 -> MATLAB Function/9(bt0)
  Constant4/1 -> MATLAB Function/10(g0)
  Constant5/1 -> MATLAB Function/1(xt0)
  vt0/1 -> MATLAB Function/2(vt0)
  w0/1 -> MATLAB Function/4(w0)
  ddx_td/1 -> Gain/1
  Gain/1 -> Atan/1
  l_h/1 -> MATLAB Function/8(l0)
  Atan/1 -> Sum1/2
  MATLAB Function/1(Kp) -> Product1/1  "Kp"
  Sum1/1 -> Discrete Derivative1/1, Product1/2
  Ftw0/1 -> MATLAB Function/5(Ftw0)
  Theta/1 -> Sum1/1, MATLAB Function/3(th0)
  Product1/1 -> Sum11/1

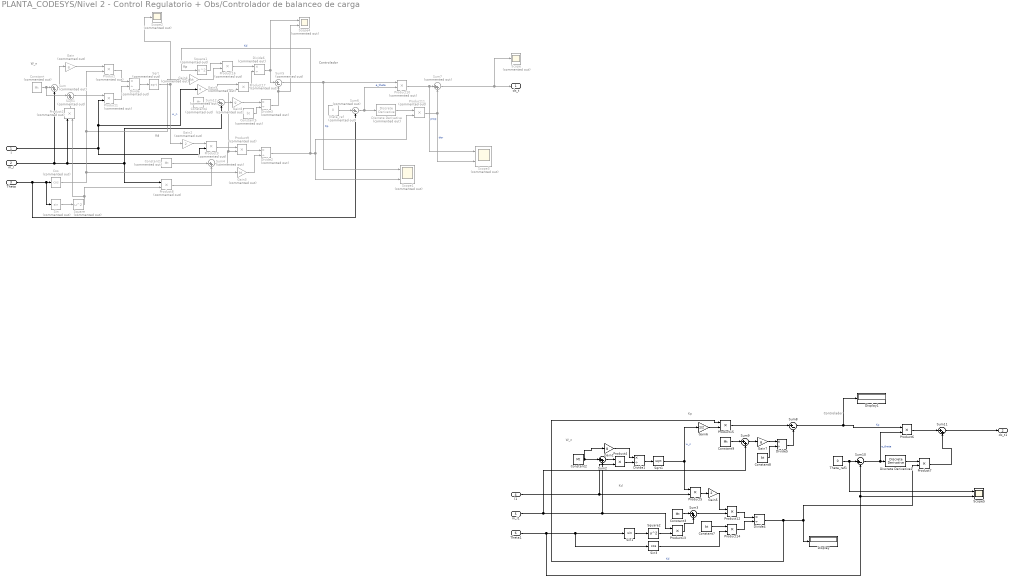
== system PLANTA_CODESYS/Nivel 2 - Control Regulatorio + Obs/Controlador de balanceo de carga ==
  note: Kp
  note: W_n
  note: Controlador
  note: Kd
  note: W_n
  note: Controlador
  note: Kp
  note: Kd
  l : Inport
  m_l : Inport  Port=2
  Theta : Inport  Port=3
  l1 : Inport  Port=4
  m_l1 : Inport  Port=5
  Theta1 : Inport  Port=6
  Constant : Constant  Commented=on  Value=Mt
  Constant1 : Constant  Commented=on  Value=Mt
  Constant2 : Constant  Value=Mt
  Constant3 : Constant  Value=Mt
  Constant4 : Constant  Commented=on  Value=Mt
  Constant5 : Constant  Commented=on  Value=bt
  Constant7 : Constant  Value=bt
  Constant8 : Constant  Value=bt
  Constant9 : Constant  Value=Mt
  Cos : Trigonometry  Commented=on  Operator=cos
  Discrete Derivative : simulink/Discrete/Discrete Derivative  Commented=on  gainval=1/T_s2  ICPrevScaledInput=0.0  OutMin=[]  OutMax=[]  OutDataType=fixdt(1, 16)  OutScaling=2^-10  DoSatur=off
  Discrete Derivative1 : simulink/Discrete/Discrete Derivative  gainval=1.0  ICPrevScaledInput=0.0  OutMin=[]  OutMax=[]  OutDataType=fixdt(1, 16)  OutScaling=2^-10  DoSatur=off
  Display : Display
  Display1 : Display
  Divide{,2..3,6} (4 alike) : Product  Commented=on  Inputs=*/
  Divide1 : Product  Inputs=*/
  Divide4 : Product  Inputs=*/
  Divide5 : Product  Inputs=*/
  Gain : Gain  Commented=on  Gain=g
  Gain1 : Gain  Gain=g
  Gain2 : Gain  Commented=on  Gain=2
  Gain3 : Gain  Commented=on  Gain=bt
  Gain4 : Gain  Commented=on  Gain=bt
  Gain5 : Gain  Gain=2
  Gain6 : Gain  Gain=1/2
  Gain7 : Gain  Gain=g
  Gain8 : Gain  Commented=on  Gain=g
  Gain9 : Gain  Commented=on  Gain=4
  Product{,1..3,8..11,16..17} (10 alike) : Product  Commented=on
  Product{4..7,12..15} (8 alike) : Product
  Scope : Scope  Commented=on
  Scope1 : Scope  Commented=on  NumInputPorts=2
  Scope2 : Scope  Commented=on
  Scope3 : Scope  Commented=on  NumInputPorts=2
  Scope4 : Scope  Commented=on  NumInputPorts=2
  Scope5 : Scope  NumInputPorts=2
  Sin : Trigonometry  Commented=on
  Sin1 : Trigonometry
  Sin3 : Trigonometry  Operator=cos
  Sqrt : Sqrt  Commented=on
  Sqrt1 : Sqrt
  Square : Math  Commented=on  Operator=square
  Square1 : Math  Commented=on  Operator=square
  Square2 : Math  Operator=square
  Sum{,1,4,7,12} (5 alike) : Sum  Commented=on  Inputs=|++
  Sum10 : Sum  Inputs=|+-
  Sum{2..3,9,11} (4 alike) : Sum  Inputs=|++
  Sum5 : Sum  Commented=on  Inputs=|+-
  Sum6 : Sum  Commented=on  Inputs=|+-
  Sum8 : Sum  Inputs=|+-
  Theta_ref : Constant  Commented=on  Value=0
  Theta_ref1 : Constant  Value=0
  dx_t : Outport
  dx_t1 : Outport  Port=2
  wires:
  Theta_ref/1 -> Sum6/1
  Sum6/1 -> Product10/2, Discrete Derivative/1  "e_theta"
  Product11/1 -> Scope3/2, Sum7/2  "der"
  Divide/1 -> Sqrt/1
  Sum/1 -> Gain/1
  Theta/1 -> Sin/1, Cos/1, Sum6/2
  m_l/1 -> Sum/2, Product8/1, Sum12/2, Product2/1
  Product10/1 -> Scope3/1, Sum7/1  "prop"
  Product/1 -> Divide/1
  Product15/1 -> Sum8/1
  Gain1/1 -> Divide1/1
  Constant3/1 -> Sum3/1
  Product14/1 -> Divide4/2
  Sin3/1 -> Product14/2
  Product4/1 -> Divide1/2
  Divide5/1 -> Sum8/2
  Sum8/1 -> Display1/1, Product6/1  "Kp"
  Constant9/1 -> Sum9/1
  Sqrt1/1 -> Product5/1, Gain6/1  "w_n"
  Sum2/1 -> Product4/1
  Theta_ref1/1 -> Scope5/1, Sum10/1
  Sin1/1 -> Square2/1
  Sum11/1 -> dx_t1/1
  Constant8/1 -> Divide5/2
  Sum9/1 -> Gain7/1
  Constant2/1 -> Gain1/1, Sum2/1
  Constant7/1 -> Product14/1
  Product5/1 -> Gain5/1
  Theta1/1 -> Sin3/1, Sin1/1, Scope5/2, Sum10/2
  l1/1 -> Product4/2, Product5/2
  Gain7/1 -> Divide5/1
  Sum10/1 -> Product6/2, Discrete Derivative1/1  "e_theta"
  Gain6/1 -> Product15/2
  Divide4/1 -> Product7/2, Display/1, Product15/1  "Kd"
  Discrete Derivative1/1 -> Product7/1
  Gain5/1 -> Product12/1
  Square2/1 -> Product13/2
  Product12/1 -> Divide4/1
  m_l1/1 -> Product13/1, Sum2/2, Sum9/2
  Product7/1 -> Sum11/2
  Product13/1 -> Sum3/2
  Sum3/1 -> Product12/2
  Product6/1 -> Sum11/1
  Divide1/1 -> Sqrt1/1
  Constant/1 -> Sum1/1, Sum/1
  Sin/1 -> Square/1
  Cos/1 -> Gain4/1, Product/2, Gain3/1
  Gain/1 -> Product/1
  l/1 -> Gain9/1, Product1/2, Product3/2
  Sum1/1 -> Product1/1
  Product2/1 -> Sum1/2
  Square/1 -> Product8/2, Product2/2
  Product1/1 -> Divide/2
  Sqrt/1 -> Scope2/1, Gain2/1  "w_n"
  Gain2/1 -> Product3/1
  Constant1/1 -> Sum4/1
  Product8/1 -> Sum4/2
  Sum4/1 -> Product9/2, Product17/2
  Product3/1 -> Product9/1
  Product9/1 -> Divide2/1
  Gain3/1 -> Divide2/2
  Divide2/1 -> Square1/1, Product11/2, Scope1/2  "Kd"
  Constant4/1 -> Sum12/1
  Sum12/1 -> Gain8/1
  Gain8/1 -> Divide3/1
  Divide3/1 -> Scope4/2, Sum5/2
  Sum5/1 -> Scope1/1, Product10/1  "Kp"
  Sum7/1 -> dx_t/1, Scope/1
  Constant5/1 -> Divide3/2
  Discrete Derivative/1 -> Product11/1
  Gain4/1 -> Product16/2
  Square1/1 -> Product16/1
  Product16/1 -> Divide6/1
  Gain9/1 -> Product17/1
  Product17/1 -> Divide6/2
  Divide6/1 -> Scope4/1, Sum5/1

== system PLANTA_CODESYS/Nivel 2 - Control Regulatorio + Obs/Controlador de balanceo1 ==
  note: Controlador
  ml : Inport
  l_h : Inport  Port=2
  theta : Inport  Port=3
  dx_t : Inport  Port=4
  ddx_t_ref : Inport  Port=5
  Atan : Trigonometry  Operator=atan
  Discrete Derivative : simulink/Discrete/Discrete Derivative  gainval=1.0  ICPrevScaledInput=0.0  OutMin=[]  OutMax=[]  OutDataType=fixdt(1, 16)  OutScaling=2^-10  DoSatur=off
  Display : Display
  Display1 : Display
  Gain : Gain  Gain=-1/g
  Gain Scheduling Kd : Lookup_n-D  NumberOfTableDimensions=3  BreakpointsForDimension1=ml_breakpoints  BreakpointsForDimension2=l_breakpoints  BreakpointsForDimension3=at_breakpoints  BreakpointsForDimension4=at_breakpoints  Table=Kd_table  InterpMethod=Flat  ExtrapMethod=Clip  InternalRulePriority=Speed  RndMeth=Simplest
      settings: InputPortMap=u0,u1,u2
  Gain Scheduling Kp : Lookup_n-D  NumberOfTableDimensions=3  BreakpointsForDimension1=ml_breakpoints  BreakpointsForDimension2=at_breakpoints  BreakpointsForDimension3=l_breakpoints  BreakpointsForDimension4=at_breakpoints  Table=Kp_table  InterpMethod=Flat  ExtrapMethod=Clip  InternalRulePriority=Speed  RndMeth=Simplest
      settings: InputPortMap=u0,u1,u2
  Product1 : Product
  Product7 : Product
  Scope1 : Scope  NumInputPorts=2
  Sum1 : Sum  Inputs=|-+
  Sum11 : Sum  Inputs=|++
  vel_bal* : Outport
  wires:
  Discrete Derivative/1 -> Product7/1
  Gain Scheduling Kd/1 -> Product7/2, Display/1  "Kd"
  Gain/1 -> Atan/1
  Gain Scheduling Kp/1 -> Display1/1, Product1/1  "Kp"
  theta/1 -> Scope1/1, Sum1/1  "theta"
  Product1/1 -> Sum11/1
  Atan/1 -> Scope1/2, Sum1/2  "ref"
  Product7/1 -> Sum11/2
  ddx_t_ref/1 -> Gain Scheduling Kd/3, Gain Scheduling Kp/3, Gain/1
  Sum1/1 -> Discrete Derivative/1, Product1/2  "e_tita"
  Sum11/1 -> vel_bal*/1  "vel_bal"
  ml/1 -> Gain Scheduling Kd/1, Gain Scheduling Kp/1
  l_h/1 -> Gain Scheduling Kd/2, Gain Scheduling Kp/2

== system PLANTA_CODESYS/Nivel 2 - Control Regulatorio + Obs/Controlador de izaje ==
  dl_href : Inport
  dl_h : Inport  Port=2
  Gain : Gain  Gain=T_s2/2
  Gain1 : Gain  Gain=K_hsia
  Gain2 : Gain  Gain=b_ha
  Gain3 : Gain  Gain=T_s2/2
  Gain8 : Gain  Gain=K_hsa
  Scope : Scope
  Sum : Sum  Inputs=|+-
  Sum{1..4} (4 alike) : Sum  Inputs=|++
  Sum5 : Sum  Inputs=+|+|+
  Unit Delay{,1..3} (4 alike) : UnitDelay  SampleTime=T_s2  HasFrameUpgradeWarning=on
  T_hm* : Outport
  wires:
  Gain2/1 -> Sum5/3
  Unit Delay1/1 -> Sum2/2  "Ik-1"
  Unit Delay3/1 -> Sum4/2  "Ik-1"
  dl_h/1 -> Sum/2
  Unit Delay/1 -> Sum1/2  "d_ek-1"
  Gain/1 -> Sum2/1  "Ik"
  Gain3/1 -> Sum4/1  "Ik"
  Sum5/1 -> T_hm*/1
  dl_href/1 -> Sum/1
  Gain1/1 -> Sum5/1
  Sum/1 -> Gain2/1, Unit Delay/1, Sum1/1, Scope/1  "d_ek"
  Sum4/1 -> Unit Delay3/1, Gain1/1
  Unit Delay2/1 -> Sum3/2  "ek-1"
  Sum3/1 -> Gain3/1
  Sum2/1 -> Sum3/1, Unit Delay2/1, Gain8/1, Unit Delay1/1  "ek"
  Gain8/1 -> Sum5/2
  Sum1/1 -> Gain/1

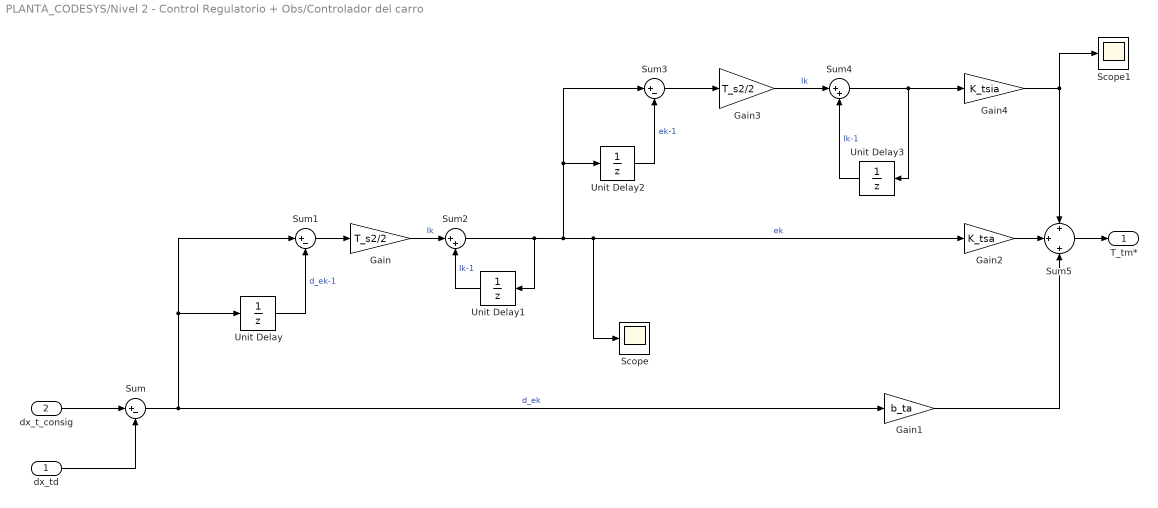
== system PLANTA_CODESYS/Nivel 2 - Control Regulatorio + Obs/Controlador del carro ==
  dx_td : Inport
  dx_t_consig : Inport  Port=2
  Gain : Gain  Gain=T_s2/2
  Gain1 : Gain  Gain=b_ta
  Gain2 : Gain  Gain=K_tsa
  Gain3 : Gain  Gain=T_s2/2
  Gain4 : Gain  Gain=K_tsia
  Scope : Scope
  Scope1 : Scope
  Sum : Sum  Inputs=|+-
  Sum1 : Sum  Inputs=|+-
  Sum2 : Sum  Inputs=|++
  Sum3 : Sum  Inputs=|+-
  Sum4 : Sum  Inputs=|++
  Sum5 : Sum  Inputs=+|+|+
  Unit Delay{,1..3} (4 alike) : UnitDelay  SampleTime=T_s2  HasFrameUpgradeWarning=on
  T_tm* : Outport
  wires:
  Unit Delay3/1 -> Sum4/2  "Ik-1"
  Unit Delay2/1 -> Sum3/2  "ek-1"
  Sum/1 -> Gain1/1, Unit Delay/1, Sum1/1  "d_ek"
  dx_t_consig/1 -> Sum/1
  Gain3/1 -> Sum4/1  "Ik"
  Sum5/1 -> T_tm*/1
  dx_td/1 -> Sum/2
  Sum1/1 -> Gain/1
  Unit Delay/1 -> Sum1/2  "d_ek-1"
  Sum2/1 -> Unit Delay1/1, Sum3/1, Unit Delay2/1, Scope/1, Gain2/1  "ek"
  Gain/1 -> Sum2/1  "Ik"
  Gain2/1 -> Sum5/2
  Sum3/1 -> Gain3/1
  Unit Delay1/1 -> Sum2/2  "Ik-1"
  Sum4/1 -> Gain4/1, Unit Delay3/1
  Gain1/1 -> Sum5/3
  Gain4/1 -> Scope1/1, Sum5/1

== system PLANTA_CODESYS/Nivel 2 - Control Regulatorio + Obs/Controlador del carro1 ==
  dx_td : Inport
  dx_t_consig : Inport  Port=2
  Gain : Gain  Gain=T_s2/2
  Gain1 : Gain  Gain=b_ta
  Gain2 : Gain  Gain=K_tsa
  Gain3 : Gain  Gain=T_s2/2
  Gain4 : Gain  Gain=K_tsia
  Scope : Scope
  Scope1 : Scope
  Sum : Sum  Inputs=|+-
  Sum1 : Sum  Inputs=|+-
  Sum2 : Sum  Inputs=|++
  Sum3 : Sum  Inputs=|+-
  Sum4 : Sum  Inputs=|++
  Sum5 : Sum  Inputs=+|+|+
  Unit Delay{,1..3} (4 alike) : UnitDelay  SampleTime=T_s2  HasFrameUpgradeWarning=on
  T_tm* : Outport
  wires:
  Unit Delay3/1 -> Sum4/2  "Ik-1"
  Unit Delay2/1 -> Sum3/2  "ek-1"
  Sum/1 -> Gain1/1, Unit Delay/1, Sum1/1  "d_ek"
  dx_t_consig/1 -> Sum/1
  Gain3/1 -> Sum4/1  "Ik"
  Sum5/1 -> T_tm*/1
  dx_td/1 -> Sum/2
  Sum1/1 -> Gain/1
  Unit Delay/1 -> Sum1/2  "d_ek-1"
  Sum2/1 -> Unit Delay1/1, Sum3/1, Unit Delay2/1, Scope/1, Gain2/1  "ek"
  Gain/1 -> Sum2/1  "Ik"
  Gain2/1 -> Sum5/2
  Sum3/1 -> Gain3/1
  Unit Delay1/1 -> Sum2/2  "Ik-1"
  Sum4/1 -> Gain4/1, Unit Delay3/1
  Gain1/1 -> Sum5/3
  Gain4/1 -> Scope1/1, Sum5/1

== system PLANTA_CODESYS/Nivel 2 - Control Regulatorio + Obs/Modulador de torque Motor - Izaje ==
  T_hm* : Inport
  State-Space : StateSpace  A=A_hm  B=B_hm  C=C_hm  D=D_hm  InitialCondition=0
  T_hm : Outport
  wires:
  T_hm*/1 -> State-Space/1
  State-Space/1 -> T_hm/1

== system PLANTA_CODESYS/Nivel 2 - Control Regulatorio + Obs/Modulador torque Motor - Carro ==
  T_tm* : Inport
  State-Space : StateSpace  A=A_tm  B=B_tm  C=C_tm  D=D_tm  InitialCondition=0
  T_tm : Outport
  wires:
  State-Space/1 -> T_tm/1
  T_tm*/1 -> State-Space/1

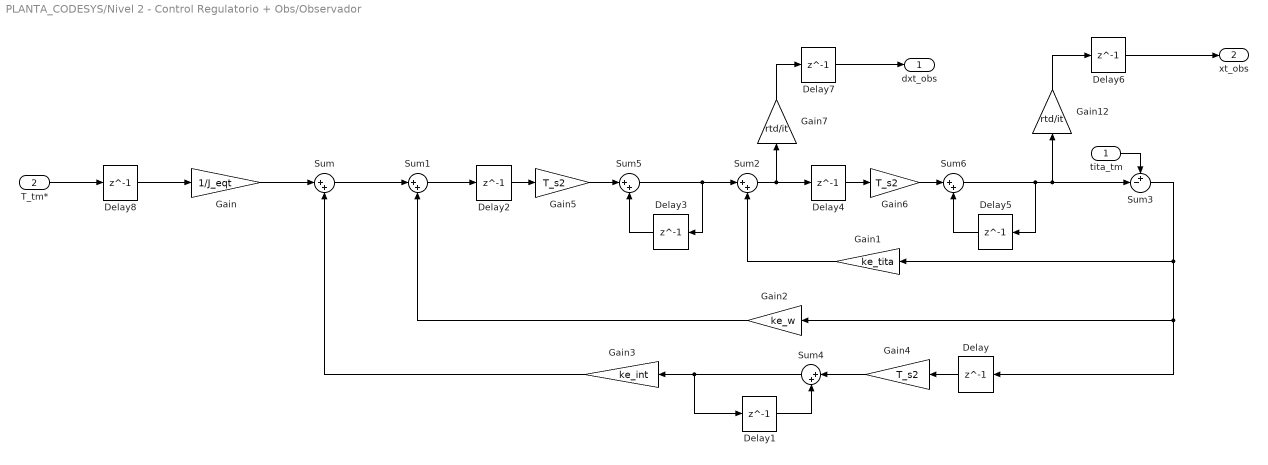
== system PLANTA_CODESYS/Nivel 2 - Control Regulatorio + Obs/Observador ==
  tita_tm : Inport
  T_tm* : Inport  Port=2
  Delay : Delay  DelayLength=1  InitialCondition=0  InputProcessing=Columns as channels (frame based)  SampleTime=T_s2
  Delay{1..5,8} (6 alike) : Delay  DelayLength=1  InputProcessing=Columns as channels (frame based)  SampleTime=T_s2
  Delay6 : Delay  DelayLength=1  InitialCondition=-20  InputProcessing=Columns as channels (frame based)  SampleTime=T_s2
  Delay7 : Delay  DelayLength=1  InitialCondition=0  InputProcessing=Columns as channels (frame based)  SampleTime=T_s2
  Gain : Gain  Gain=1/J_eqt
  Gain1 : Gain  Gain=ke_tita
  Gain12 : Gain  Gain=rtd/it
  Gain2 : Gain  Gain=ke_w
  Gain3 : Gain  Gain=ke_int
  Gain4 : Gain  Gain=T_s2
  Gain5 : Gain  Gain=T_s2
  Gain6 : Gain  Gain=T_s2
  Gain7 : Gain  Gain=rtd/it
  Sum{,1..2,4..6} (6 alike) : Sum  Inputs=|++
  Sum3 : Sum  Inputs=+-|
  dxt_obs : Outport
  xt_obs : Outport  Port=2
  wires:
  T_tm*/1 -> Delay8/1
  Gain/1 -> Sum/1
  Sum/1 -> Sum1/1
  Sum1/1 -> Delay2/1
  Sum5/1 -> Delay3/1, Sum2/1
  Sum2/1 -> Gain7/1, Delay4/1
  Sum6/1 -> Gain12/1, Sum3/2, Delay5/1
  tita_tm/1 -> Sum3/1
  Sum3/1 -> Gain2/1, Delay/1, Gain1/1
  Gain1/1 -> Sum2/2
  Gain2/1 -> Sum1/2
  Gain3/1 -> Sum/2
  Delay/1 -> Gain4/1
  Gain4/1 -> Sum4/1
  Delay1/1 -> Sum4/2
  Sum4/1 -> Gain3/1, Delay1/1
  Delay3/1 -> Sum5/2
  Delay2/1 -> Gain5/1
  Gain5/1 -> Sum5/1
  Delay5/1 -> Sum6/2
  Delay4/1 -> Gain6/1
  Gain6/1 -> Sum6/1
  Gain7/1 -> Delay7/1
  Gain12/1 -> Delay6/1
  Delay6/1 -> xt_obs/1
  Delay7/1 -> dxt_obs/1
  Delay8/1 -> Gain/1

== system PLANTA_CODESYS/Nivel 2 - Control Regulatorio + Obs1/Controlador de balanceo1 ==
  note: Controlador
  ml : Inport
  l_h : Inport  Port=2
  theta : Inport  Port=3
  ddx_t : Inport  Port=4
  ddx_t_ref : Inport  Port=5
  Atan : Trigonometry  Operator=atan
  Discrete Derivative : simulink/Discrete/Discrete Derivative  gainval=1.0  ICPrevScaledInput=0.0  OutMin=[]  OutMax=[]  OutDataType=fixdt(1, 16)  OutScaling=2^-10  DoSatur=off
  Gain : Gain  Gain=-1/g
  Gain Scheduling Kd : Lookup_n-D  NumberOfTableDimensions=3  BreakpointsForDimension1=ml_breakpoints  BreakpointsForDimension2=l_breakpoints  BreakpointsForDimension3=at_breakpoints  BreakpointsForDimension4=at_breakpoints  Table=Kd_table  InterpMethod=Flat  ExtrapMethod=Clip  InternalRulePriority=Speed  RndMeth=Simplest
      settings: InputPortMap=u0,u1,u2
  Gain Scheduling Kp : Lookup_n-D  NumberOfTableDimensions=3  BreakpointsForDimension1=ml_breakpoints  BreakpointsForDimension2=l_breakpoints  BreakpointsForDimension3=at_breakpoints  BreakpointsForDimension4=at_breakpoints  Table=Kp_table  InterpMethod=Flat  ExtrapMethod=Clip  InternalRulePriority=Speed  RndMeth=Simplest
      settings: InputPortMap=u0,u1,u2
  Gain1 : Gain  Gain=0.3
  Gain2 : Gain  Gain=-0.3
  Product1 : Product
  Product7 : Product
  Scope1 : Scope  NumInputPorts=2
  Sum1 : Sum  Inputs=|-+
  Sum11 : Sum  Inputs=|++
  vel_bal* : Outport
  wires:
  Discrete Derivative/1 -> Product7/1
  Gain Scheduling Kd/1 -> Gain2/1  "Kd"
  Gain/1 -> Atan/1
  Gain Scheduling Kp/1 -> Gain1/1  "Kp"
  theta/1 -> Discrete Derivative/1, Scope1/1, Sum1/1  "theta"
  Atan/1 -> Scope1/2, Sum1/2  "ref"
  Product7/1 -> Sum11/2
  ddx_t_ref/1 -> Gain/1
  Sum1/1 -> Product1/2  "e_tita"
  Sum11/1 -> vel_bal*/1  "vel_bal"
  ml/1 -> Gain Scheduling Kd/1, Gain Scheduling Kp/1
  l_h/1 -> Gain Scheduling Kd/2, Gain Scheduling Kp/2
  Gain1/1 -> Product1/1
  Gain2/1 -> Product7/2
  ddx_t/1 -> Gain Scheduling Kp/3, Gain Scheduling Kd/3
  Product1/1 -> Sum11/1

== system PLANTA_CODESYS/Nivel 2 - Control Regulatorio + Obs1/Controlador de izaje ==
  dl_href : Inport
  dl_h : Inport  Port=2
  Discrete-Time Integrator : DiscreteIntegrator  SampleTime=T_s2  ICPrevOutput=DiscIntNeverNeededParam  ICPrevScaledInput=DiscIntNeverNeededParam
  Discrete-Time Integrator1 : DiscreteIntegrator  SampleTime=T_s2  ICPrevOutput=DiscIntNeverNeededParam  ICPrevScaledInput=DiscIntNeverNeededParam
  Gain1 : Gain  Gain=K_hsia
  Gain2 : Gain  Gain=b_ha
  Gain8 : Gain  Gain=K_hsa
  Sum : Sum  Inputs=|+-
  Sum5 : Sum  Inputs=+|+|+
  T_hm* : Outport
  wires:
  Gain2/1 -> Sum5/3
  dl_h/1 -> Sum/2
  Sum5/1 -> T_hm*/1
  dl_href/1 -> Sum/1
  Gain1/1 -> Sum5/1
  Sum/1 -> Gain2/1, Discrete-Time Integrator/1  "d_ek"
  Gain8/1 -> Sum5/2
  Discrete-Time Integrator/1 -> Gain8/1, Discrete-Time Integrator1/1
  Discrete-Time Integrator1/1 -> Gain1/1

== system PLANTA_CODESYS/Nivel 2 - Control Regulatorio + Obs1/Controlador del carro1 ==
  dx_td : Inport
  dx_t_consig : Inport  Port=2
  Discrete-Time Integrator : DiscreteIntegrator  SampleTime=T_s2  ICPrevOutput=DiscIntNeverNeededParam  ICPrevScaledInput=DiscIntNeverNeededParam
  Discrete-Time Integrator1 : DiscreteIntegrator  SampleTime=T_s2  ICPrevOutput=DiscIntNeverNeededParam  ICPrevScaledInput=DiscIntNeverNeededParam
  Gain1 : Gain  Gain=b_ta
  Gain2 : Gain  Gain=K_tsa
  Gain4 : Gain  Gain=K_tsia
  Sum : Sum  Inputs=|+-
  Sum5 : Sum  Inputs=+|+|+
  T_tm* : Outport
  wires:
  Sum/1 -> Gain1/1, Discrete-Time Integrator/1  "d_ek"
  dx_t_consig/1 -> Sum/1
  Sum5/1 -> T_tm*/1
  dx_td/1 -> Sum/2
  Gain2/1 -> Sum5/2
  Gain1/1 -> Sum5/3
  Gain4/1 -> Sum5/1
  Discrete-Time Integrator/1 -> Gain2/1, Discrete-Time Integrator1/1
  Discrete-Time Integrator1/1 -> Gain4/1

== system PLANTA_CODESYS/Nivel 2 - Control Regulatorio + Obs1/Modulador de torque Motor - Izaje ==
  T_hm* : Inport
  State-Space : StateSpace  A=A_hm  B=B_hm  C=C_hm  D=D_hm  InitialCondition=0
  T_hm : Outport
  wires:
  T_hm*/1 -> State-Space/1
  State-Space/1 -> T_hm/1

== system PLANTA_CODESYS/Nivel 2 - Control Regulatorio + Obs1/Modulador torque Motor - Carro ==
  T_tm* : Inport
  State-Space : StateSpace  A=A_tm  B=B_tm  C=C_tm  D=D_tm  InitialCondition=0
  T_tm : Outport
  wires:
  State-Space/1 -> T_tm/1
  T_tm*/1 -> State-Space/1

== system PLANTA_CODESYS/Nivel 2 - Control Regulatorio + Obs1/Observador_Control_Posicion ==
  T_tm* : Inport
  x_td_real : Inport  Port=2
  x_t_ref : Inport  Port=3
  theta_l : Inport  Port=4
  F_hw : Inport  Port=5
  Discrete Derivative : simulink/Discrete/Discrete Derivative  gainval=1.0  ICPrevScaledInput=0.0  OutMin=[]  OutMax=[]  OutDataType=fixdt(1, 16)  OutScaling=2^-10  DoSatur=off
  Fuerzas de tension de cable en Carro : Subsystem
  Observador : Subsystem
  Subsystem : Subsystem
  Traslacion del carro : Subsystem
  ddx_t_obs : Outport
  dx_t_pos : Outport  Port=2
  dx_td_obs : Outport  Port=3
  wires:
  Observador/1(dx_td_obs) -> Fuerzas de tension de cable en Carro/2(dx_td), dx_td_obs/1  "dx_td_obs"
  x_td_real/1 -> Fuerzas de tension de cable en Carro/1(x_td), Observador/1(x_td)
  x_t_ref/1 -> Subsystem/2(xt_ref)
  Subsystem/1(dxt_pos) -> dx_t_pos/1
  Traslacion del carro/1(x_t) -> Fuerzas de tension de cable en Carro/3(x_t), Subsystem/1(xt_obs)  "x_t_obs"
  Traslacion del carro/2(dx_t) -> Fuerzas de tension de cable en Carro/4(dx_t), Discrete Derivative/1  "dx_t_obs"
  theta_l/1 -> Traslacion del carro/3(theta_l)
  F_hw/1 -> Traslacion del carro/2(F_hw)
  Fuerzas de tension de cable en Carro/1(F_tw) -> Traslacion del carro/1(F_tw)
  T_tm*/1 -> Observador/2(T_tm*)
  Discrete Derivative/1 -> ddx_t_obs/1

== system PLANTA_CODESYS/PLANTA/Accionamiento de Izaje ==
  T_hm : Inport
  F_hw : Inport  Port=2
  BRK_h : Inport  Port=3
  BRK_hE : Inport  Port=4
  Add : Sum  Inputs=+++-
  Freno : Subsystem
  Freno Emergencia : Subsystem
  Gain : Gain  Gain=rhd
  Gain1 : Gain  Gain=ih
  Gain2 : Gain  Gain=(2*bhd+2*bhm*(ih)^2)/rhd
  Gain3 : Gain  Gain=-2/rhd
  Gain4 : Gain  Gain=ih
  Gain6 : Gain  Gain=-rhd/(2*Jhd_hEb+2*Jhm_hb*(ih)^2)
  Integrator : Integrator  InitialCondition=l_h_ini
  Integrator1 : Integrator  InitialCondition=dl_h_ini
  Scope : Scope
  Sum : Sum  Inputs=-|+||
  l_h : Outport
  dl_h : Outport  Port=2
  wires:
  Gain1/1 -> Add/2
  Integrator1/1 -> dl_h/1, Integrator/1, Gain3/1, Gain2/1
  F_hw/1 -> Gain/1
  Gain6/1 -> Scope/1, Integrator1/1  "ddl_h"
  T_hm/1 -> Sum/2
  Freno Emergencia/1(T_hEB) -> Add/3
  BRK_hE/1 -> Freno Emergencia/2(BRK_hE)
  Gain4/1 -> Freno/1(w_hm)  "w_hm"
  Gain/1 -> Add/4
  Integrator/1 -> l_h/1
  Gain3/1 -> Freno Emergencia/1(w_hd), Gain4/1  "w_hd"
  Sum/1 -> Gain1/1
  Add/1 -> Gain6/1
  Freno/1(T_hb) -> Sum/1
  Gain2/1 -> Add/1
  BRK_h/1 -> Freno/2(BRK_h)

== system PLANTA_CODESYS/PLANTA/Accionamiento del carro ==
  F_tw : Inport
  BRK_t : Inport  Port=2
  T_tm : Inport  Port=3
  Constant : Constant  Value=0
  Gain : Gain  Gain=rtd
  Gain1 : Gain  Gain=it
  Gain2 : Gain  Gain=(btm*(it)^2+btd)/rtd
  Gain3 : Gain  Gain=rtd/(Jtd+Jtm_tb*(it)^2)
  Gain4 : Gain  Gain=-(btd*it)/rtd
  Integrator : Integrator  InitialCondition=dx_td_ini
  Integrator1 : Integrator  InitialCondition=x_td_ini
  Saturation : Saturate  UpperLimit=Ttb_Max  LowerLimit=-Ttb_Max
  Sum : Sum  Inputs=|++
  Sum1 : Sum  Inputs=-|+|-
  Switch : Switch  Criteria=u2 > Threshold  SaturateOnIntegerOverflow=off  InputSameDT=off
  x_td : Outport
  dx_td : Outport  Port=2
  ddx_td : Outport  Port=3
  wires:
  Integrator/1 -> Gain4/1, dx_td/1, Integrator1/1, Gain2/1
  Gain4/1 -> Saturation/1
  T_tm/1 -> Sum/2
  Constant/1 -> Switch/1
  Gain/1 -> Sum1/1
  Saturation/1 -> Switch/3
  Gain3/1 -> ddx_td/1, Integrator/1  "ddx_td"
  BRK_t/1 -> Switch/2
  Sum1/1 -> Gain3/1
  Switch/1 -> Sum/1  "T_tb"
  F_tw/1 -> Gain/1
  Gain1/1 -> Sum1/2
  Integrator1/1 -> x_td/1
  Gain2/1 -> Sum1/3
  Sum/1 -> Gain1/1
